simulink model "buck_nncontroller_3_50"  (R2021a)
settings: Solver=VariableStepAuto  StartTime=0.0  StopTime=10.0  RelTol=1e-3
libraries: neural x155
(part 8 of 8)

== system buck_nncontroller_3_50/Feed-Forward Neural Network/Layer 4/Delays 1 ==
  "p{4}" : Inport  PortDimensions=50
      mask Display: e = 0.06;c1 = [120 230 180]/255;c2 = ([120 230 180]+0)/(256+128);c3 = ([120 230 180]+128)/(256+128);patch([0 1 1 0],[0 0 1 1],c1);patch([0 1 1 1-e 1-e 0+e],[0 0 1 1-e 0+e 0+e],c2);patch([0 0 1 1-e 0+e 0+e],[0 1 1 1-e 1-e 0+e],c3);plot([0 1 1 0 0],[0 0 1 1 0]);
  mux : Mux  Inputs=1
      mask Display: e = 0.06;c1 = [120 150 230]/255;c2 = ([120 150 230]+0)/383;c3 = ([120 150 230]+128)/383;patch([0 1 1 0],[0 0 1 1],c1);patch([0 1 1 1-e 1-e 0+e],[0 0 1 1-e 0+e 0+e],c2);patch([0 0 1 1-e 0+e 0+e],[0 1 1 1-e 1-e 0+e],c3);plot([0 1 1 0 0],[0 0 1 1 0]);disp('Mux')
  "pd{4,3}" : Outport
      mask Display: e = 0.06;c1 = [120 230 180]/255;c2 = ([120 230 180]+0)/(256+128);c3 = ([120 230 180]+128)/(256+128);patch([0 1 1 0],[0 0 1 1],c1);patch([0 1 1 1-e 1-e 0+e],[0 0 1 1-e 0+e 0+e],c2);patch([0 0 1 1-e 0+e 0+e],[0 1 1 1-e 1-e 0+e],c3);plot([0 1 1 0 0],[0 0 1 1 0]);
  wires:
  "p{4}"/1 -> mux/1
  mux/1 -> "pd{4,3}"/1

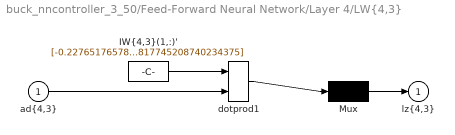
== system buck_nncontroller_3_50/Feed-Forward Neural Network/Layer 4/LW{4,3} ==
  "ad{4,3}" : Inport  PortDimensions=50
      mask Display: e = 0.06;c1 = [120 230 180]/255;c2 = ([120 230 180]+0)/(256+128);c3 = ([120 230 180]+128)/(256+128);patch([0 1 1 0],[0 0 1 1],c1);patch([0 1 1 1-e 1-e 0+e],[0 0 1 1-e 0+e 0+e],c2);patch([0 0 1 1-e 0+e 0+e],[0 1 1 1-e 1-e 0+e],c3);plot([0 1 1 0 0],[0 0 1 1 0]);
  "IW{4,3}(1,:)'" : Constant  Value=[-0.2276517657857584087111035842099227011203765869140625;0.59757188101541791613868781496421433985233306884765625;-0.56971772601384318424067032538005150854587554931640625;0.9333700543535801141814545189845375716686248779296875;-0.967253639421925104358024327666498720645904541015625;0.90817604612558000543032221685280092060565948486328125;0.376403017201153600179708291761926375329494476318359375;-0.184770461732487845107897328489343635737895965576171875;0.7323037567538086545226860835100524127483367919921875;-0.0786097394173504160352905500985798425972461700439453125;0.628803624188658094595893999212421476840972900390625;-0.1518194448839414179008855398933519609272480010986328125;0.1670979374189636990077900691176182590425014495849609375;0.64649741968244234247009671889827586710453033447265625;0.1271395133437760449623965541832149028778076171875;0.90868489340213376426191871360060758888721466064453125;0.2446990706523315406428764617885462939739227294921875;0.54602826147903460451971113798208534717559814453125;0.189381474388951975829087359670666046440601348876953125;0.56694170857404646568511452642269432544708251953125;0.373902134793886065100565474494942463934421539306640625;-0.1998496014183117619467111580888740718364715576171875;0.167752861627278371248195298903738148510456085205078125;0.2353043294305210419992135939537547528743743896484375;0.731551209149066128389904406503774225711822509765625;0.0132931838407162050685883514233864843845367431640625;-0.136017266945551551504678400306147523224353790283203125;-0.0161722507960651018521502919611521065235137939453125;0.0827168685329839892261816203244961798191070556640625;0.826207767327247655231303724576719105243682861328125;-1.076905725557440351991544957854785025119781494140625;0.90136116388333931137566423785756342113018035888671875;-0.78781146309583738318593759686336852610111236572265625;0.72164161616405009258556901841075159609317779541015625;-0.203690199300754326561246898563695140182971954345703125;0.574201789294199738122870257939212024211883544921875;0.7822975062056063411120021555689163506031036376953125;0.369550786684152310357376336469314992427825927734375;-0.0020891296509983853062208947193312269519083201885223388671875;-0.4667780995780070885103896216605789959430694580078125;0.454348779345947473284894613243523053824901580810546875;0.8989218281577844305019198145600967109203338623046875;0.2614082803512129959955245794844813644886016845703125;0.6452476923824550514297015979536809027194976806640625;-0.7332591907821335297512632678262889385223388671875;-0.2315638685963075094065288794809021055698394775390625;0.48664516355372910982879375296761281788349151611328125;0.396878455351755754509923690420691855251789093017578125;0.95273695689772741612699746838188730180263519287109375;0.6360529951568716366949729490443132817745208740234375]
      mask Display: e = 0.06;c1 = [120 150 230]/255;c2 = ([120 150 230]+0)/383;c3 = ([120 150 230]+128)/383;patch([0 1 1 0],[0 0 1 1],c1);patch([0 1 1 1-e 1-e 0+e],[0 0 1 1-e 0+e 0+e],c2);patch([0 0 1 1-e 0+e 0+e],[0 1 1 1-e 1-e 0+e],c3);plot([0 1 1 0 0],[0 0 1 1 0]);disp('weights');
  Mux : Mux  Inputs=1
      mask Display: e = 0.06;c1 = [120 150 230]/255;c2 = ([120 150 230]+0)/383;c3 = ([120 150 230]+128)/383;patch([0 1 1 0],[0 0 1 1],c1);patch([0 1 1 1-e 1-e 0+e],[0 0 1 1-e 0+e 0+e],c2);patch([0 0 1 1-e 0+e 0+e],[0 1 1 1-e 1-e 0+e],c3);plot([0 1 1 0 0],[0 0 1 1 0]);disp('Mux');
  dotprod1 : neural/Weight Functions/dotprod
  "lz{4,3}" : Outport
      mask Display: e = 0.06;c1 = [120 230 180]/255;c2 = ([120 230 180]+0)/(256+128);c3 = ([120 230 180]+128)/(256+128);patch([0 1 1 0],[0 0 1 1],c1);patch([0 1 1 1-e 1-e 0+e],[0 0 1 1-e 0+e 0+e],c2);patch([0 0 1 1-e 0+e 0+e],[0 1 1 1-e 1-e 0+e],c3);plot([0 1 1 0 0],[0 0 1 1 0]);
  wires:
  "IW{4,3}(1,:)'"/1 -> dotprod1/1
  "ad{4,3}"/1 -> dotprod1/2
  dotprod1/1 -> Mux/1
  Mux/1 -> "lz{4,3}"/1
